simulink model "Model_Automatique"  (R2020a)
settings: Solver=VariableStepAuto  StartTime=0.0  StopTime=10.0  RelTol=1e-3
values from neighbouring files (symbols this model uses):
  Kh = 2*Ubat    (= 48)    [Simulation_Trottinette.m]    (also in Simulation_Trottinette_BF.m)
  L = 2e-3    (= 0.002)    [Simulation_Trottinette.m]    (also in Simulation_Trottinette_BF.m)
  R = 1    [Simulation_Trottinette.m]    (also in Simulation_Trottinette_BF.m)
settings Model: Creator=mdescham  LastModifiedBy=mdescham

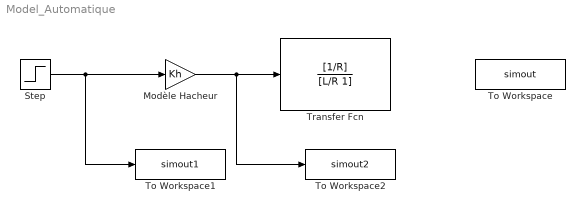
== system Model_Automatique ==
  Modèle Hacheur : Gain  Gain=Kh
  Step : Step  SampleTime=0
  To Workspace : ToWorkspace  VariableName=simout  SaveFormat=Timeseries  SampleTime=-1
  To Workspace1 : ToWorkspace  VariableName=simout1  SaveFormat=Timeseries  SampleTime=-1
  To Workspace2 : ToWorkspace  VariableName=simout2  SaveFormat=Timeseries  SampleTime=-1
  Transfer Fcn : TransferFcn  Numerator=[1/R]  Denominator=[L/R 1]
  wires:
  Step/1 -> Modèle Hacheur/1, To Workspace1/1
  Modèle Hacheur/1 -> To Workspace2/1, Transfer Fcn/1
